simulink model "smc2"  (R2020a)
settings: Solver=VariableStepAuto  StartTime=0.0  StopTime=10.0  RelTol=1e-3
settings Model: Creator=khoi  LastModifiedBy=khoi

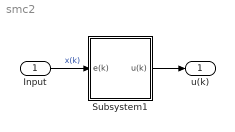
== system smc2 ==
  Input : Inport
  Subsystem1 : Subsystem  mask{A=0, B=0, C=0, q=0, T=0, lam=0, gamm=0, vphi=0, bet=0}
      mask prompts: A "A discrete"; B "B discrete"; C "C sliding param"; q "convergence gain >0"; T "sample time"; lam "lambda > 0"; gamm "gamma > 0"; vphi "varphi > 0"; bet "0< beta <1"
      mask DialogControl ParameterGroupVar Prompt: State
      mask DialogControl ParameterGroupVar_copy Prompt: Exponential term
  u(k) : Outport
  wires:
  Subsystem1/1(u(k)) -> u(k)/1
  Input/1 -> Subsystem1/1(e(k))  "x(k)"

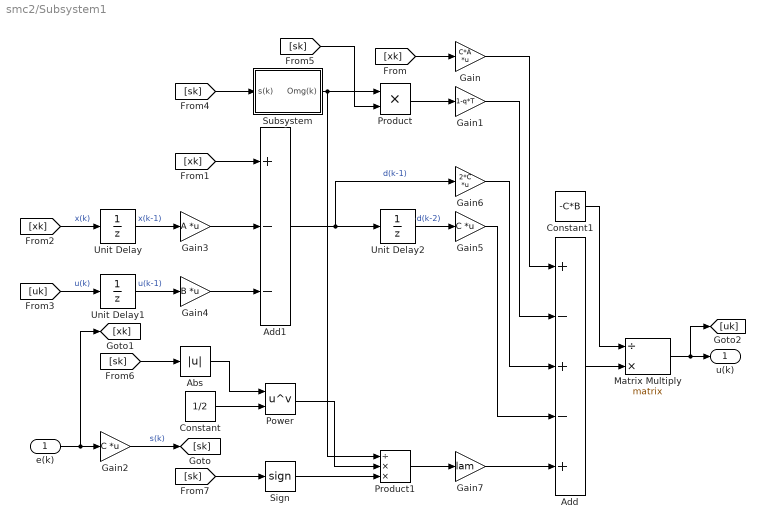
== system smc2/Subsystem1 ==
  e(k) : Inport
  Abs : Abs
  Add : Sum  Inputs=+-+-+
  Add1 : Sum  Inputs=+--
  Constant : Constant  Value=1/2
  Constant1 : Constant  Value=-C*B
  Gain : Gain  Gain=C*A  Multiplication=Matrix(K*u) (u vector)
  Gain1 : Gain  Gain=1-q*T
  Gain2 : Gain  Gain=C  Multiplication=Matrix(K*u) (u vector)
  Gain3 : Gain  Gain=A  Multiplication=Matrix(K*u) (u vector)
  Gain4 : Gain  Gain=B  Multiplication=Matrix(K*u) (u vector)
  Gain5 : Gain  Gain=C  Multiplication=Matrix(K*u) (u vector)
  Gain6 : Gain  Gain=2*C  Multiplication=Matrix(K*u) (u vector)
  Gain7 : Gain  Gain=lam
  Matrix Multiply : Product  Inputs=/*  Multiplication=Matrix(*)
  Power : Math  Operator=pow  SaturateOnIntegerOverflow=on
  Product : Product
  Product1 : Product  Inputs=/**
  Sign : Signum
  Subsystem : Subsystem
  Unit Delay : UnitDelay  SampleTime=-1  HasFrameUpgradeWarning=on
  Unit Delay1 : UnitDelay  SampleTime=-1  HasFrameUpgradeWarning=on
  Unit Delay2 : UnitDelay  SampleTime=-1  HasFrameUpgradeWarning=on
  u(k) : Outport
  wires:
  Product1/1 -> Gain7/1
  Gain4/1 -> Add1/3
  Gain5/1 -> Add/4
  Abs/1 -> Power/1
  [sk] -> Subsystem/1(s(k))
  Add1/1 -> Unit Delay2/1, Gain6/1  "d(k-1)"
  Gain3/1 -> Add1/2
  [xk] -> Gain/1
  Gain1/1 -> Add/2
  [sk] -> Abs/1
  [xk] -> Unit Delay/1  "x(k)"
  Product/1 -> Gain1/1
  Unit Delay/1 -> Gain3/1  "x(k-1)"
  Sign/1 -> Product1/3
  [sk] -> Sign/1
  Subsystem/1(Omg(k)) -> Product/1, Product1/1
  [uk] -> Unit Delay1/1  "u(k)"
  Constant/1 -> Power/2
  Gain7/1 -> Add/5
  Add/1 -> Matrix Multiply/2
  Unit Delay1/1 -> Gain4/1  "u(k-1)"
  Constant1/1 -> Matrix Multiply/1
  [xk] -> Add1/1
  [sk] -> Product/2
  Unit Delay2/1 -> Gain5/1  "d(k-2)"
  Power/1 -> Product1/2
  Gain6/1 -> Add/3
  Gain/1 -> Add/1
  Gain2/1 -> [sk]  "s(k)"
  Matrix Multiply/1 -> u(k)/1, [uk]
  e(k)/1 -> Gain2/1, [xk]

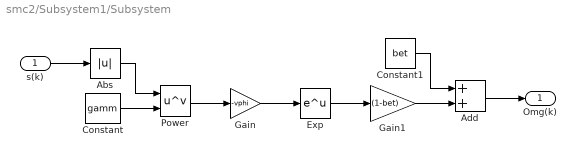
== system smc2/Subsystem1/Subsystem ==
  s(k) : Inport
  Abs : Abs
  Add : Sum
  Constant : Constant  Value=gamm
  Constant1 : Constant  Value=bet
  Exp : Math  SaturateOnIntegerOverflow=on
  Gain : Gain  Gain=-vphi
  Gain1 : Gain  Gain=(1-bet)
  Power : Math  Operator=pow  SaturateOnIntegerOverflow=on
  Omg(k) : Outport
  wires:
  Constant/1 -> Power/2
  Power/1 -> Gain/1
  s(k)/1 -> Abs/1
  Exp/1 -> Gain1/1
  Abs/1 -> Power/1
  Gain1/1 -> Add/2
  Constant1/1 -> Add/1
  Gain/1 -> Exp/1
  Add/1 -> Omg(k)/1
